simulink model "OCRe"  (Simulink 8.5)
settings: Solver=ode23t  SolverMode=SingleTasking  StartTime=0.0  StopTime=0.5  FixedStep=1e-5  MaxStep=0.7e-4  RelTol=1e-3  AbsTol=1e-2
libraries: powerlib x35, powerlib_extras x3
settings Model: Creator=azadpour  LastModifiedBy=PC  ExtModeTrigMode=oneshot  ExtModeArmWhenConnect=off
settings DataIOCC: LimitDataPoints=off
settings OptimizationCC: BlockReduction=off  BooleanDataType=off  InitFltsAndDblsToZero=on
settings DebuggingCC: SaveWithParameterizedLinksMsg=none  SignalResolutionControl=TryResolveAllWithWarning  MultiTaskDSMMsg=warning  MultiTaskCondExecSysMsg=none  FcnCallInpInsideContextMsg=UseLocalSettings
settings HardwareCC: TargetUnknown=on
settings GRTTargetCC: TargetFcnLib=ansi_tfl_tmw.mat

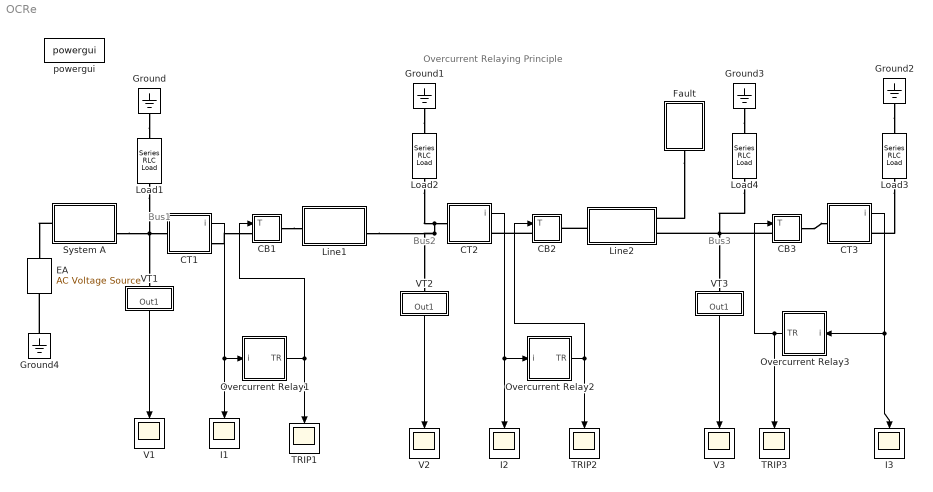
== system OCRe ==
  note: Overcurrent Relaying Principle
  note: Bus3
  note: Bus2
  note: Bus1
  " Load2" : powerlib/Elements/Series RLC Load  LConnTagsString=a  RConnTagsString=__new0  NominalVoltage=138e3  NominalFrequency=60  ActivePower=100e6  InductivePower=30e6  CapacitivePower=0  Setx0=off  InitialVoltage=0  SetiL0=off  InitialCurrent=0  Measurements=None
  " Load3" : powerlib/Elements/Series RLC Load  LConnTagsString=a  RConnTagsString=__new0  NominalVoltage=138e3  NominalFrequency=60  ActivePower=50e6  InductivePower=15e6  CapacitivePower=0  Setx0=off  InitialVoltage=0  SetiL0=off  InitialCurrent=0  Measurements=None
  " Load4" : powerlib/Elements/Series RLC Load  LConnTagsString=a  RConnTagsString=__new0  NominalVoltage=138e3  NominalFrequency=60  ActivePower=50e6  InductivePower=15e6  CapacitivePower=0  Setx0=off  InitialVoltage=0  SetiL0=off  InitialCurrent=0  Measurements=None
  CB1 : Subsystem  mask(CB){t_op=15}
      mask prompts: t_op "Operating time [ms]"
      mask Display: disp('CB')
  CB2 : Subsystem  mask(CB){t_op=15}
      mask prompts: t_op "Operating time [ms]"
      mask Display: disp('CB')
  CB3 : Subsystem  mask(CB){t_op=25}
      mask prompts: t_op "Operating time [ms]"
      mask Display: disp('CB')
  CT1 : Subsystem  mask(CT){Prim=1600, Sec=1}
      mask prompts: Prim "Primary Current [A]"; Sec "Secondary Current [A]"
      mask Display: disp('CT')
  CT2 : Subsystem  mask(CT){Prim=1000, Sec=1}
      mask prompts: Prim "Primary Current [A]"; Sec "Secondary Current [A]"
      mask Display: disp('CT')
  CT3 : Subsystem  mask(CT){Prim=500, Sec=1}
      mask prompts: Prim "Primary Current [A]"; Sec "Secondary Current [A]"
      mask Display: disp('CT')
  EA : powerlib/Electrical Sources/AC Voltage Source  Amplitude=158000  Phase=0  Frequency=60  SampleTime=0  Measurements=None
  Fault : Subsystem  mask(Fault){RF=0, tf=0.02}
      mask prompts: RF "Resistance [ohm]"; tf "Time [sec]"
      mask Display: plot(0,0,100,100,[44,47,56,38,50],[23,8,64,44,97],[56,47],[25,8])
  Ground{,1..4} (5 alike) : powerlib/Elements/Ground  LConnTagsString=a
  I1 : Scope
      settings: TickLabels=on  YMin=-0.00501  YMax=-0.00489
  I2 : Scope
      settings: TickLabels=on  YMin=-0.04  YMax=0.04
  I3 : Scope
      settings: TickLabels=on  YMin=-0.7  YMax=0.7
  Line1 : Subsystem  mask(Simple Line){R=2, X=20, p=0.5}
      mask prompts: R "Resistance [ohm]"; X "Reactance [ohm]"; p "Fault location [pu]"
      mask init:
      | R1=R*p; R2=R*(1-p);
      | L1=X*p/(2*pi*60);L2=X*(1-p)/(2*pi*60);
  Line2 : Subsystem  mask(Simple Line){R=2, X=20, p=0.5}
      mask prompts: R "Resistance [ohm]"; X "Reactance [ohm]"; p "Fault location [pu]"
      mask init:
      | R1=R*p; R2=R*(1-p);
      | L1=X*p/(2*pi*60);L2=X*(1-p)/(2*pi*60);
  Load1 : powerlib/Elements/Series RLC Load  LConnTagsString=a  RConnTagsString=__new0  NominalVoltage=138e3  NominalFrequency=60  ActivePower=100e6  InductivePower=30e6  CapacitivePower=0  Setx0=off  InitialVoltage=0  SetiL0=off  InitialCurrent=0  Measurements=None
  Overcurrent Relay1 : Subsystem
  Overcurrent Relay2 : Subsystem
  Overcurrent Relay3 : Subsystem
  System A : Subsystem  mask(Simple Line){R=1, X=10, p=0.5}
      mask prompts: R "Resistance [ohm]"; X "Reactance [ohm]"; p "Fault location [pu]"
      mask init:
      | R1=R*p; R2=R*(1-p);
      | L1=X*p/(2*pi*60);L2=X*(1-p)/(2*pi*60);
  TRIP1 : Scope
      settings: TickLabels=on  YMin=-1  YMax=1
  TRIP2 : Scope
      settings: TickLabels=on  YMin=-1  YMax=1
  TRIP3 : Scope
      settings: TickLabels=on  YMin=-1  YMax=1
  V1 : Scope
      settings: TickLabels=on  YMin=-175000  YMax=175000
  V2 : Scope
      settings: TickLabels=on  YMin=-15000  YMax=15000
  V3 : Scope
      settings: TickLabels=on  YMin=-125000  YMax=125000
  VT1 : Subsystem  mask(VT){vol1=138, vol2=100}
      mask prompts: vol1 "Primary voltage [kV]"; vol2 "Secondary voltage [V]"
      mask Display: disp('VT')
  VT2 : Subsystem  mask(VT){vol1=138, vol2=100}
      mask prompts: vol1 "Primary voltage [kV]"; vol2 "Secondary voltage [V]"
      mask Display: disp('VT')
  VT3 : Subsystem  mask(VT){vol1=138, vol2=100}
      mask prompts: vol1 "Primary voltage [kV]"; vol2 "Secondary voltage [V]"
      mask Display: disp('VT')
  powergui : powerlib/powergui  SimulationMode=Continuous  SolverType=Tustin/Backward Euler (TBE)  SampleTime=0  frequency=60  SPID=off  DisableSnubberDevices=off  DisableRonSwitches=off  DisableVfSwitches=off  SwTol=0  DisplayEquations=off  Interpol=off  methode=off  Ts=0  FunctionMessages=off  echomessages=off  HookPort=off  EnableUseOfTLC=off  x0status=blocks  frequencyindice=60  Pbase=100e6  ErrMax=1e-4  Iterations=50  UnitsV=kV  UnitsW=MW  buscounter=0  RestoreLinks=warning  ResistiveCurrentMeasurement=off  Frange=[0:2:500]  Ylog=off  Xlog=on  ShowGrid=off  save=off  variable=ZData  structure=0  ZoomFFT=on  StartTime=0.0  cycles=1  DisplayStyle=1  fundamental=60  FreqAxis=off  MaxFrequency=1000  frequencyindicesteady=1  RmsSteady=1  display=off
  wires:
  VT1/1(Out1) -> V1/1
  Overcurrent Relay1/1(TR) -> TRIP1/1, CB1/1(T)
  Overcurrent Relay2/1(TR) -> TRIP2/1, CB2/1(T)
  VT3/1(Out1) -> V3/1
  Overcurrent Relay3/1(TR) -> CB3/1(T), TRIP3/1
  VT2/1(Out1) -> V2/1
  CT1/1(i) -> I1/1, Overcurrent Relay1/1(i)
  CT2/1(i) -> I2/1, Overcurrent Relay2/1(i)
  CT3/1(i) -> Overcurrent Relay3/1(i), I3/1
  connections:
  Ground/LConn1 -- Load1/LConn1
  Ground1/LConn1 -- " Load2"/LConn1
  Fault/LConn1 -- Line2/RConn1
  System A/LConn1 -- EA/RConn1
  Ground4/LConn1 -- EA/LConn1
  Load1/RConn1 -- CT1/LConn1 -- VT1/LConn1 -- System A/RConn2
  CT1/RConn1 -- CB1/LConn1
  CB1/RConn1 -- Line1/LConn1
  CT2/LConn1 -- Line1/RConn2 -- VT2/LConn1 -- " Load2"/RConn1
  CB2/LConn1 -- CT2/RConn1
  Line2/LConn1 -- CB2/RConn1
  CB3/LConn1 -- " Load4"/RConn1 -- Line2/RConn2 -- VT3/LConn1
  " Load3"/RConn1 -- CT3/RConn1
  Ground2/LConn1 -- " Load3"/LConn1
  CB3/RConn1 -- CT3/LConn1
  Ground3/LConn1 -- " Load4"/LConn1

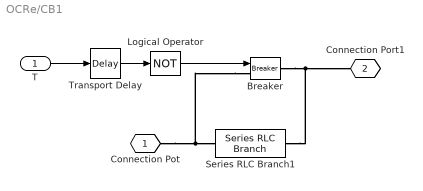
== system OCRe/CB1 ==
  T : Inport
  Breaker : powerlib/Elements/Breaker  Tag=PoWeRsYsTeMbLoCk  InitialState=0  SwitchingTimes="[ 1/60  5/60 ]"  External=on  BreakerResistance=0.01  SnubberResistance=1e6  SnubberCapacitance=inf  Measurements=None  MoreParameters=off  NoBreakLoop=off
  Logical Operator : Logic  Operator=NOT  Inputs=1
  Series RLC Branch1 : powerlib/Elements/Series RLC Branch  LConnTagsString=__new0  RConnTagsString=__new0  BranchType=RLC  Resistance=1  Inductance=1e-3  SetiL0=off  InitialCurrent=0  Capacitance=1e-6  Setx0=off  InitialVoltage=0  Measurements=None
  Transport Delay : TransportDelay  DelayTime=t_op/1000
  Connection Pot : PMIOPort  Tag=PMCPort  Port=1  Side=Left
  Connection Port1 : PMIOPort  Tag=PMCPort  Port=2  Side=Right
  wires:
  Logical Operator/1 -> Breaker/1
  Transport Delay/1 -> Logical Operator/1
  T/1 -> Transport Delay/1
  connections:
  Series RLC Branch1/RConn1 -- Connection Port1/RConn1 -- Breaker/RConn1
  Breaker/LConn1 -- Series RLC Branch1/LConn1 -- Connection Pot/RConn1

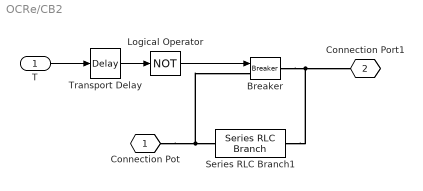
== system OCRe/CB2 ==
  T : Inport
  Breaker : powerlib/Elements/Breaker  Tag=PoWeRsYsTeMbLoCk  InitialState=0  SwitchingTimes="[ 1/60  5/60 ]"  External=on  BreakerResistance=0.01  SnubberResistance=1e6  SnubberCapacitance=inf  Measurements=None  MoreParameters=off  NoBreakLoop=off
  Logical Operator : Logic  Operator=NOT  Inputs=1
  Series RLC Branch1 : powerlib/Elements/Series RLC Branch  LConnTagsString=__new0  RConnTagsString=__new0  BranchType=RLC  Resistance=1  Inductance=1e-3  SetiL0=off  InitialCurrent=0  Capacitance=1e-6  Setx0=off  InitialVoltage=0  Measurements=None
  Transport Delay : TransportDelay  DelayTime=t_op/1000
  Connection Pot : PMIOPort  Tag=PMCPort  Port=1  Side=Left
  Connection Port1 : PMIOPort  Tag=PMCPort  Port=2  Side=Right
  wires:
  T/1 -> Transport Delay/1
  Transport Delay/1 -> Logical Operator/1
  Logical Operator/1 -> Breaker/1
  connections:
  Connection Pot/RConn1 -- Series RLC Branch1/LConn1 -- Breaker/LConn1
  Breaker/RConn1 -- Connection Port1/RConn1 -- Series RLC Branch1/RConn1

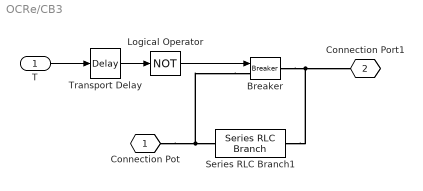
== system OCRe/CB3 ==
  T : Inport
  Breaker : powerlib/Elements/Breaker  Tag=PoWeRsYsTeMbLoCk  InitialState=0  SwitchingTimes="[ 1/60  5/60 ]"  External=on  BreakerResistance=0.01  SnubberResistance=1e6  SnubberCapacitance=inf  Measurements=None  MoreParameters=off  NoBreakLoop=off
  Logical Operator : Logic  Operator=NOT  Inputs=1
  Series RLC Branch1 : powerlib/Elements/Series RLC Branch  LConnTagsString=__new0  RConnTagsString=__new0  BranchType=RLC  Resistance=1  Inductance=1e-3  SetiL0=off  InitialCurrent=0  Capacitance=1e-6  Setx0=off  InitialVoltage=0  Measurements=None
  Transport Delay : TransportDelay  DelayTime=t_op/1000
  Connection Pot : PMIOPort  Tag=PMCPort  Port=1  Side=Left
  Connection Port1 : PMIOPort  Tag=PMCPort  Port=2  Side=Right
  wires:
  Logical Operator/1 -> Breaker/1
  Transport Delay/1 -> Logical Operator/1
  T/1 -> Transport Delay/1
  connections:
  Series RLC Branch1/RConn1 -- Connection Port1/RConn1 -- Breaker/RConn1
  Breaker/LConn1 -- Series RLC Branch1/LConn1 -- Connection Pot/RConn1

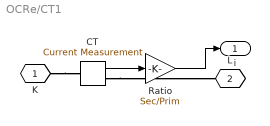
== system OCRe/CT1 ==
  CT : powerlib/Measurements/Current Measurement  PhasorSimulation=off  OutputType=Complex  PSBequivalent=0
  Ratio : Gain  Gain=Sec/Prim  SaturateOnIntegerOverflow=on  OutDataTypeStr=Inherit: Same as input  ParamDataTypeStr=Inherit: Same as input
  K : PMIOPort  Tag=PMCPort  Port=1  Side=Left
  L : PMIOPort  Tag=PMCPort  Port=2  Side=Right
  i : Outport  InitialOutput=0
  wires:
  Ratio/1 -> i/1
  CT/1 -> Ratio/1
  connections:
  CT/RConn1 -- L/RConn1
  K/RConn1 -- CT/LConn1

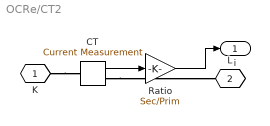
== system OCRe/CT2 ==
  CT : powerlib/Measurements/Current Measurement  PhasorSimulation=off  OutputType=Complex  PSBequivalent=0
  Ratio : Gain  Gain=Sec/Prim  SaturateOnIntegerOverflow=on  OutDataTypeStr=Inherit: Same as input  ParamDataTypeStr=Inherit: Same as input
  K : PMIOPort  Tag=PMCPort  Port=1  Side=Left
  L : PMIOPort  Tag=PMCPort  Port=2  Side=Right
  i : Outport  InitialOutput=0
  wires:
  CT/1 -> Ratio/1
  Ratio/1 -> i/1
  connections:
  K/RConn1 -- CT/LConn1
  CT/RConn1 -- L/RConn1

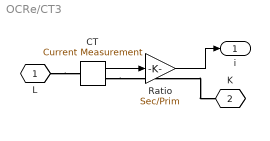
== system OCRe/CT3 ==
  CT : powerlib/Measurements/Current Measurement  PhasorSimulation=off  OutputType=Complex  PSBequivalent=0
  Ratio : Gain  Gain=Sec/Prim  SaturateOnIntegerOverflow=on  OutDataTypeStr=Inherit: Same as input  ParamDataTypeStr=Inherit: Same as input
  L : PMIOPort  Tag=PMCPort  Port=1  Side=Left
  K : PMIOPort  Tag=PMCPort  Port=2  Side=Right
  i : Outport  InitialOutput=0
  wires:
  Ratio/1 -> i/1
  CT/1 -> Ratio/1
  connections:
  CT/RConn1 -- K/RConn1
  L/RConn1 -- CT/LConn1

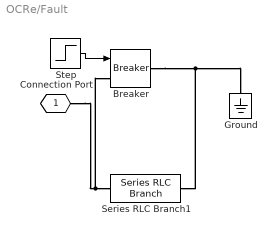
== system OCRe/Fault ==
  Breaker : powerlib/Elements/Breaker  Tag=PoWeRsYsTeMbLoCk  InitialState=0  SwitchingTimes="[ 1/60  5/60 ]"  External=on  BreakerResistance=0.01  SnubberResistance=1e6  SnubberCapacitance=inf  Measurements=None  MoreParameters=off  NoBreakLoop=off
  Ground : powerlib/Elements/Ground  LConnTagsString=a
  Series RLC Branch1 : powerlib/Elements/Series RLC Branch  LConnTagsString=__new0  RConnTagsString=__new0  BranchType=RLC  Resistance=1  Inductance=1e-3  SetiL0=off  InitialCurrent=0  Capacitance=1e-6  Setx0=off  InitialVoltage=0  Measurements=None
  Step : Step  Time=tf
  Connection Port : PMIOPort  Tag=PMCPort  Port=1  Side=Left
  wires:
  Step/1 -> Breaker/1
  connections:
  Series RLC Branch1/LConn1 -- Breaker/LConn1 -- Connection Port/RConn1
  Series RLC Branch1/RConn1 -- Ground/LConn1 -- Breaker/RConn1

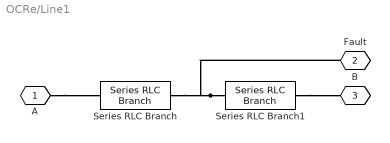
== system OCRe/Line1 ==
  Series RLC Branch : powerlib/Elements/Series RLC Branch  LConnTagsString=__new0  RConnTagsString=__new0  BranchType=RL  Resistance=R1  Inductance=L1  SetiL0=off  InitialCurrent=0  Capacitance=1.0  Setx0=off  InitialVoltage=0  Measurements=None
  Series RLC Branch1 : powerlib/Elements/Series RLC Branch  LConnTagsString=__new0  RConnTagsString=__new0  BranchType=RL  Resistance=R2  Inductance=L2  SetiL0=off  InitialCurrent=0  Capacitance=1.0  Setx0=off  InitialVoltage=0  Measurements=None
  A : PMIOPort  Tag=PMCPort  Port=1  Side=Left
  Fault : PMIOPort  Tag=PMCPort  Port=2  Side=Right
  B : PMIOPort  Tag=PMCPort  Port=3  Side=Right
  connections:
  Series RLC Branch1/RConn1 -- B/RConn1
  Series RLC Branch1/LConn1 -- Series RLC Branch/RConn1 -- Fault/RConn1
  A/RConn1 -- Series RLC Branch/LConn1

== system OCRe/Line2 ==
  Series RLC Branch : powerlib/Elements/Series RLC Branch  LConnTagsString=__new0  RConnTagsString=__new0  BranchType=RL  Resistance=R1  Inductance=L1  SetiL0=off  InitialCurrent=0  Capacitance=1.0  Setx0=off  InitialVoltage=0  Measurements=None
  Series RLC Branch1 : powerlib/Elements/Series RLC Branch  LConnTagsString=__new0  RConnTagsString=__new0  BranchType=RL  Resistance=R2  Inductance=L2  SetiL0=off  InitialCurrent=0  Capacitance=1.0  Setx0=off  InitialVoltage=0  Measurements=None
  A : PMIOPort  Tag=PMCPort  Port=1  Side=Left
  Fault : PMIOPort  Tag=PMCPort  Port=2  Side=Right
  B : PMIOPort  Tag=PMCPort  Port=3  Side=Right
  connections:
  A/RConn1 -- Series RLC Branch/LConn1
  Series RLC Branch1/LConn1 -- Fault/RConn1 -- Series RLC Branch/RConn1
  Series RLC Branch1/RConn1 -- B/RConn1

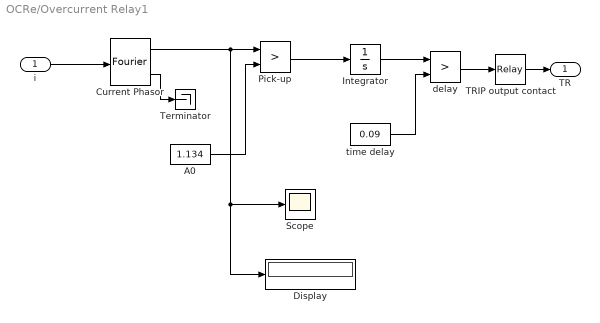
== system OCRe/Overcurrent Relay1 ==
  i : Inport
  A0 : Constant  Value=1.134
  Current Phasor : powerlib_extras/Measurements/Fourier  f1=60  n=1
  Display : Display
  Integrator : Integrator
  Pick-up : RelationalOperator  Operator=>  InputSameDT=on
  Scope : Scope
      settings: TickLabels=on
  TRIP output contact : Relay  OnSwitchValue=0.9999  OffSwitchValue=-1
  Terminator : Terminator
  delay : RelationalOperator  Operator=>  InputSameDT=on
  time delay : Constant  Value=0.09
  TR : Outport  InitialOutput=0
  wires:
  Current Phasor/2 -> Terminator/1
  A0/1 -> Pick-up/2
  i/1 -> Current Phasor/1
  Pick-up/1 -> Integrator/1
  Integrator/1 -> delay/1
  time delay/1 -> delay/2
  delay/1 -> TRIP output contact/1
  TRIP output contact/1 -> TR/1
  Current Phasor/1 -> Pick-up/1, Scope/1, Display/1

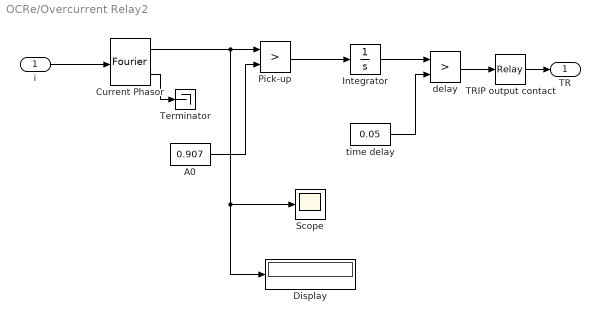
== system OCRe/Overcurrent Relay2 ==
  i : Inport
  A0 : Constant  Value=0.907
  Current Phasor : powerlib_extras/Measurements/Fourier  f1=60  n=1
  Display : Display
  Integrator : Integrator
  Pick-up : RelationalOperator  Operator=>  InputSameDT=on
  Scope : Scope
      settings: TickLabels=on
  TRIP output contact : Relay  OnSwitchValue=0.9999  OffSwitchValue=-1
  Terminator : Terminator
  delay : RelationalOperator  Operator=>  InputSameDT=on
  time delay : Constant  Value=0.05
  TR : Outport  InitialOutput=0
  wires:
  Current Phasor/1 -> Display/1, Scope/1, Pick-up/1
  TRIP output contact/1 -> TR/1
  delay/1 -> TRIP output contact/1
  time delay/1 -> delay/2
  Integrator/1 -> delay/1
  Pick-up/1 -> Integrator/1
  i/1 -> Current Phasor/1
  A0/1 -> Pick-up/2
  Current Phasor/2 -> Terminator/1

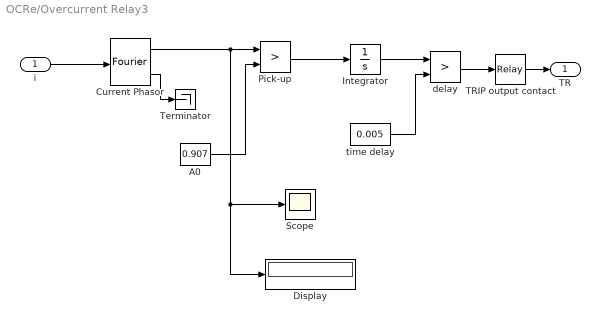
== system OCRe/Overcurrent Relay3 ==
  i : Inport
  A0 : Constant  Value=0.907
  Current Phasor : powerlib_extras/Measurements/Fourier  f1=60  n=1
  Display : Display
  Integrator : Integrator
  Pick-up : RelationalOperator  Operator=>  InputSameDT=on
  Scope : Scope
      settings: TickLabels=on
  TRIP output contact : Relay  OnSwitchValue=0.9999  OffSwitchValue=-1
  Terminator : Terminator
  delay : RelationalOperator  Operator=>  InputSameDT=on
  time delay : Constant  Value=0.005
  TR : Outport  InitialOutput=0
  wires:
  Current Phasor/2 -> Terminator/1
  A0/1 -> Pick-up/2
  i/1 -> Current Phasor/1
  Pick-up/1 -> Integrator/1
  Integrator/1 -> delay/1
  time delay/1 -> delay/2
  delay/1 -> TRIP output contact/1
  TRIP output contact/1 -> TR/1
  Current Phasor/1 -> Pick-up/1, Scope/1, Display/1

== system OCRe/System A ==
  Series RLC Branch : powerlib/Elements/Series RLC Branch  LConnTagsString=__new0  RConnTagsString=__new0  BranchType=RL  Resistance=R1  Inductance=L1  SetiL0=off  InitialCurrent=0  Capacitance=1.0  Setx0=off  InitialVoltage=0  Measurements=None
  Series RLC Branch1 : powerlib/Elements/Series RLC Branch  LConnTagsString=__new0  RConnTagsString=__new0  BranchType=RL  Resistance=R2  Inductance=L2  SetiL0=off  InitialCurrent=0  Capacitance=1.0  Setx0=off  InitialVoltage=0  Measurements=None
  A : PMIOPort  Tag=PMCPort  Port=1  Side=Left
  Fault : PMIOPort  Tag=PMCPort  Port=2  Side=Right
  B : PMIOPort  Tag=PMCPort  Port=3  Side=Right
  connections:
  A/RConn1 -- Series RLC Branch/LConn1
  Series RLC Branch1/LConn1 -- Fault/RConn1 -- Series RLC Branch/RConn1
  Series RLC Branch1/RConn1 -- B/RConn1

== system OCRe/VT1 ==
  Ground : powerlib/Elements/Ground  LConnTagsString=a
  PP : powerlib/Measurements/Voltage Measurement  Tag=PoWeRsYsTeMmEaSuReMeNt  PhasorSimulation=off  OutputType=Complex  PSBequivalent=0
  ratio : Gain  Gain=vol2/(vol1*1000)  SaturateOnIntegerOverflow=on  OutDataTypeStr=Inherit: Same as input  ParamDataTypeStr=Inherit: Same as input
  Connection Port1 : PMIOPort  Tag=PMCPort  Port=1  Side=Left
  Out1 : Outport  InitialOutput=0
  wires:
  ratio/1 -> Out1/1
  PP/1 -> ratio/1
  connections:
  Ground/LConn1 -- PP/LConn2
  Connection Port1/RConn1 -- PP/LConn1

== system OCRe/VT2 ==
  Ground : powerlib/Elements/Ground  LConnTagsString=a
  PP : powerlib/Measurements/Voltage Measurement  Tag=PoWeRsYsTeMmEaSuReMeNt  PhasorSimulation=off  OutputType=Complex  PSBequivalent=0
  ratio : Gain  Gain=vol2/(vol1*1000)  SaturateOnIntegerOverflow=on  OutDataTypeStr=Inherit: Same as input  ParamDataTypeStr=Inherit: Same as input
  Connection Port1 : PMIOPort  Tag=PMCPort  Port=1  Side=Left
  Out1 : Outport  InitialOutput=0
  wires:
  PP/1 -> ratio/1
  ratio/1 -> Out1/1
  connections:
  Connection Port1/RConn1 -- PP/LConn1
  Ground/LConn1 -- PP/LConn2

== system OCRe/VT3 ==
  Ground : powerlib/Elements/Ground  LConnTagsString=a
  PP : powerlib/Measurements/Voltage Measurement  Tag=PoWeRsYsTeMmEaSuReMeNt  PhasorSimulation=off  OutputType=Complex  PSBequivalent=0
  ratio : Gain  Gain=vol2/(vol1*1000)  SaturateOnIntegerOverflow=on  OutDataTypeStr=Inherit: Same as input  ParamDataTypeStr=Inherit: Same as input
  Connection Port1 : PMIOPort  Tag=PMCPort  Port=1  Side=Left
  Out1 : Outport  InitialOutput=0
  wires:
  ratio/1 -> Out1/1
  PP/1 -> ratio/1
  connections:
  Ground/LConn1 -- PP/LConn2
  Connection Port1/RConn1 -- PP/LConn1
